simulink model "tutorial_simplefir"  (Simulink 7.4)
settings: Solver=ode45  StartTime=0.0  StopTime=200  RelTol=1e-3
libraries: xbsIndex_r4 x7, xbsCopyrightNotice_r4 x1
settings Model: Creator=kavika  LastModifiedBy=douangp
settings DataIOCC: SignalLoggingName=sigsOut
settings OptimizationCC: InlineInvariantSignals=on  InitFltsAndDblsToZero=on
settings DebuggingCC: SaveWithParameterizedLinksMsg=none  SignalResolutionControl=TryResolveAllWithWarning  SolverPrmCheckMsg=none  MultiTaskDSMMsg=warning  MultiTaskCondExecSysMsg=none  StrictBusMsg=None
settings HardwareCC: TargetUnknown=on
settings RTWCC: IncludeERTFirstTime=on
settings GRTTargetCC: TargetFcnLib=ansi_tfl_tmw.mat

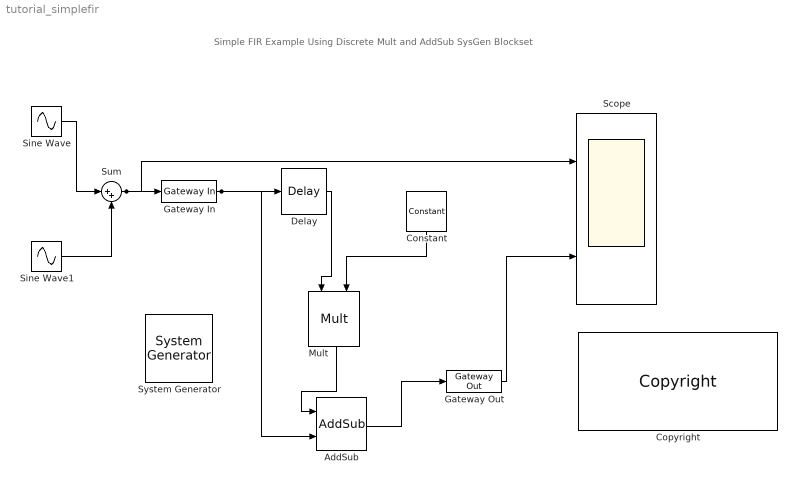
== system tutorial_simplefir ==
  note: Simple FIR Example Using Discrete
      |  Mult and AddSub SysGen Blockset
  " System Generator" : xbsIndex_r4/ System Generator  Tag=genX  SystemSampleTime=-1  xilinxfamily=spartan6  part=xc6slx16  speed=-3  package=csg324  synthesis_tool=XST  clock_wrapper=Clock Enables  directory=./netlist  testbench=off  simulink_period=1  sysclk_period=10  dcm_input_clock_period=100  incr_netlist=off  trim_vbits=Everywhere in SubSystem  dbl_ovrd=According to Block Masks  core_generation=According to Block Masks  run_coregen=off  deprecated_control=off  eval_field=0  block_type=sysgen
      settings: block_version=12.3
  AddSub : xbsIndex_r4/AddSub  mode=Addition  use_carryin=off  use_carryout=off  en=off  latency=0  precision=Full  arith_type=Unsigned  n_bits=8  bin_pt=2  quantization=Truncate  overflow=Wrap  dbl_ovrd=off  use_behavioral_HDL=on  hw_selection=Fabric  pipelined=off  use_rpm=off  block_type=addsub
      settings: xl_area=[0, 0, 0, 0, 0, 0, 0]  block_version=VER_STRING_GOES_HERE
  Constant : xbsIndex_r4/Constant  arith_type=Signed (2's comp)  const=1  n_bits=2  bin_pt=0  explicit_period=off  period=1  equ=P=C  opselect=C  inp2=PCIN>>17  opr=+  inp1=P  carry=CIN  dbl_ovrd=off  block_type=constant
      settings: block_version=VER_STRING_GOES_HERE
  Copyright : xbsCopyrightNotice_r4/Copyright  copyrighttext="Copyright (c) 2010  by  Xilinx, Inc. All rights reserved.<br><br>This file contains proprietary, confidential information of Xilinx, Inc., is distributed under licensefrom Xilinx, Inc., and may be used, copied and/or disclosed only pursuant to the terms of a valid licenseagreement with Xilinx, Inc. Xilinx hereby grants you a license to use this file solely for design,simulation, implementation and creation of design files limited to Xilinx devices or technologies. Use with non-Xilinx devices or technologies is expressly prohibited and immediately terminates your license unless covered by a separate agreement.<br><br>Xilinx is providing this design, code, or information \"as-is\" solely for use in developing programs and solutions for Xilinx devices, with no obligation on the part of Xilinx to provide support. By providingthis design, code, or information as one possible implementation of this feature, application or standard,Xilinx is making no representation that this implementation is free from any claims of infringement. Youare responsible for obtaining any rights you may require for your implementation. Xilinx expressly disclaimsany warranty whatsoever with respect to the adequacy of the implementation, including but not limited to anywarranties or representations that this implementation is free from claims of infringement, implied warrantiesof merchantability or fitness for a particular purpose.<br><br>Xilinx products are not intended for use in life support appliances, devices, or systems. Use in such applications is expressly prohibited.<br><br>Any modifications that are made to the Source Code are done at the user's sole risk and will be unsupported.<br><br>This copyright and support notice must be retained as part of this text at all times. (c) Copyright 1995-2010 Xilinx, Inc. All rights reserved."  block_type=copyright
      settings: block_version=10.1.3
      settings: infoedit=|
      | Copyright(C) 2008 by  Xilinx, Inc. All rights reserved.<br>
      | <br>
      | This file contains proprietary, confidential information of Xilinx, Inc., is distributed under license
      | from Xilinx, Inc., and may be used, copied and/or disclosed only pursuant to the terms of a valid license
      | agreement with Xilinx, Inc. Xilinx hereby grants you a license to use this file solely for design,
      | simulation, implementation and creation of design files limited to Xilinx devices or technologies. Use
      | with non-Xilinx devices or technologies is expressly prohibited and immediately terminates your license
      | unless covered by a separate agreement.<br>
      | <br>
      | Xilinx is providing this design, code, or information "as-is" solely for use in developing programs and
      | solutions for Xilinx devices, with no obligation on the part of Xilinx to provide support. By providing
      | this design, code, or information as one possible implementation of this feature, application or standard,
      | Xilinx is making no representation that this implementation is free from any claims of infringement. You
      | are responsible for obtaining any rights you may require for your implementation. Xilinx expressly disclaims
      | any warranty whatsoever with respect to the adequacy of the implementation, including but not limited to any
      | warranties or representations that this implementation is free from claims of infringement, implied warranties
      | of merchantability or fitness for a particular purpose.<br>
      | <br>
      | Xilinx products are not intended for use in life support appliances, devices, or systems. Use in such
      | applications is expressly prohibited.<br>
      | <br>
      | Any modifications that are made to the Source Code are done at the user's sole risk and will be unsupported.<br>
      | <br>
      | This copyright and support notice must be retained as part of this text at all times.
      | (c) Copyright 1995-2008 Xilinx, Inc. All rights reserved.
  Delay : xbsIndex_r4/Delay  en=off  latency=1  dbl_ovrd=off  reg_retiming=off  block_type=delay
      settings: infoedit=Hardware notes: A delay line is a chain, each link of which is an SRL16 followed by a flip-flop. If register retiming is enabled, the delay line is a chain of flip-flops.  block_version=VER_STRING_GOES_HERE
  Gateway In : xbsIndex_r4/Gateway In  arith_type="Signed  (2's comp)"  n_bits=14  bin_pt=12  quantization="Round  (unbiased: +/- Inf)"  overflow=Saturate  period=1  dbl_ovrd=off  timing_constraint=None  locs_specified=off  LOCs={}  hdl_port=on  block_type=gatewayin
      settings: infoedit="Gateway in block.  Converts inputs of type Simulink integer, double and fixed point to  Xilinx fixed point type.<P><P>Hardware notes:  In hardware these blocks become top level input ports."  xl_area=[0, 0, 0, 0, 0, 0, 0]  block_version=VER_STRING_GOES_HERE
  Gateway Out : xbsIndex_r4/Gateway Out  hdl_port=on  timing_constraint=None  locs_specified=off  LOCs={}  block_type=gatewayout
      settings: infoedit="Gateway out block.  Converts Xilinx fixed point inputs into ouputs of type Simulink integer, double, or fixed point.<P><P>Hardware notes:  In hardware these blocks become top level output ports or are discarded, depending on how they are configured."  xl_area=[0, 0, 0, 0, 0, 0, 0]  block_version=VER_STRING_GOES_HERE
  Mult : xbsIndex_r4/Mult  precision=Full  arith_type="Signed  (2's comp)"  n_bits=8  bin_pt=2  quantization=Truncate  overflow=Wrap  en=off  latency=1  dbl_ovrd=off  use_behavioral_HDL=off  opt=Speed  use_embedded=on  optimum_pipeline=off  pipeline=on  use_rpm=off  placement_style=Rectangular shape  block_type=mult
      settings: infoedit=Hardware notes: To use the internal pipeline stage of the dedicated multiplier you must select 'Pipeline to Greatest Extent Possible'.  xl_area=[0, 0, 0, 0, 0, 0, 0]  block_version=VER_STRING_GOES_HERE
  Scope : Scope  NumInputPorts=2
      settings: YMin=-1.5~-2.5  YMax=1.5~2.5
  Sine Wave : Sin  Amplitude=1  Bias=0  Frequency=.1  Phase=0  Samples=10  SampleTime=0  Offset=0
  Sine Wave1 : Sin  Amplitude=.25  Bias=0  Frequency=1.4  Phase=0  Samples=10  SampleTime=0  Offset=0
  Sum : Sum  Inputs=|++  OutDataType=sfix(16)  OutScaling=2^0  SaturateOnIntegerOverflow=on
  wires:
  Gateway In/1 -> AddSub/2, Delay/1
  Sum/1 -> Gateway In/1, Scope/1
  Gateway Out/1 -> Scope/2
  Mult/1 -> AddSub/1
  Constant/1 -> Mult/2
  AddSub/1 -> Gateway Out/1
  Sine Wave/1 -> Sum/1
  Sine Wave1/1 -> Sum/2
  Delay/1 -> Mult/1
